simulink model "Convolution_Ex2"  (R2025a)
settings: Solver=VariableStepAuto  StartTime=0.0  StopTime=128/100e6  RelTol=1e-3
undefined symbols (not defined in the file): S, Same, vsva2197, xcvc1902
libraries: aieDSP x1, vmcUtilities x1
settings Model: Creator=sdegala  LastModifiedBy=robg
settings ModelReferenceCC: EnableRefExpFcnMdlSchedulingChecks=on
settings RTWCC: GPUComputeCapability=3.5

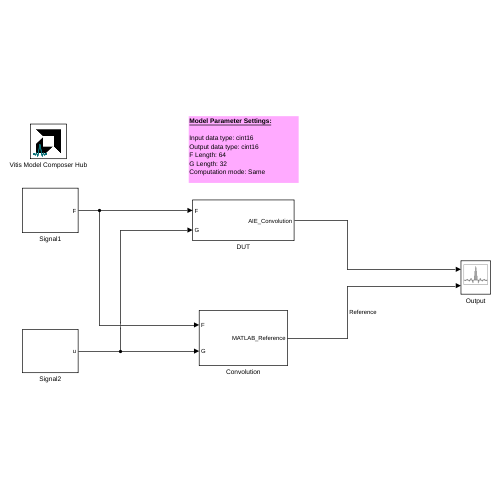
[thumbnail: Simulink's stored preview of the top-level diagram]
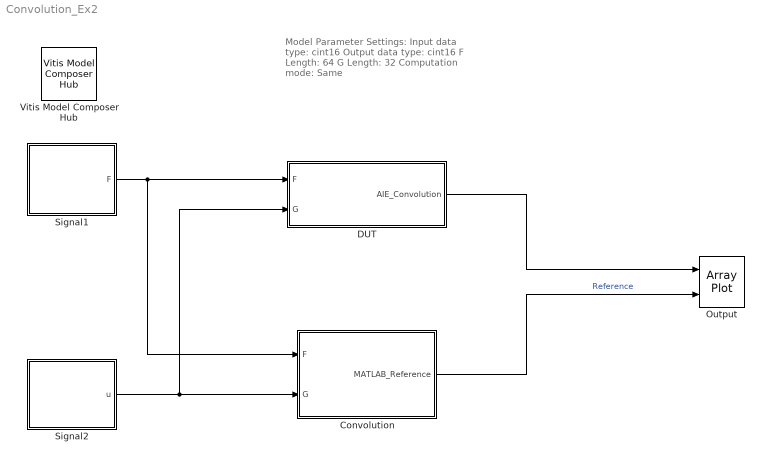
== system Convolution_Ex2 ==
  note: Model Parameter Settings:
      |
      | Input data type: cint16
      | Output data type: cint16
      | F Length: 64
      | G Length: 32
      | Computation mode: Same
  Convolution : Subsystem
  DUT : Subsystem
  Output : ArrayPlot  NumInputPorts=2  WindowPosition=[568.000000,395.000000,800.000000,500.000000,]  Visible=on  ScopeFrameLocation=window  YLimits=[-6.75 60.75]  ShowLegend=on
  Signal1 : Subsystem
  Signal2 : Subsystem
  Vitis Model Composer Hub : vmcUtilities/Vitis Model Composer Hub  Tag=genX  CodeGeneration=off  StartColumn=1  NumberOfColumns=1  TargetDirectory=./code  exportDesign=off  analyzeDesign=off  validateDesignOnHw=off  ExportType=AI Engines  IpVendor=xilinx.com  IpLibrary=hls  IpVersion=1.0  IpHWLanguage=Verilog  AieCompilerOptions={}  AieSimulatorOptions={}  CreateTestbench=off  TestbenchStackSize=10  RunRtlSim=off  RunCSim=off  RunAieSim=off  enableSimulationTimeout=on  enableGraphIterations=on  AieSimTimeout=50000  AieGraphIterations=-1  RunAieSimProfiling=off  LaunchVitisAnalyzer=off  PlotOutput=off  RunX86Sim=off  X86SimTimeout=10  GenHwImage=off  GenLibadfXo=off  GenHwValidationCode=off  PlatformType=Not Specified  HwSystemType=Baremetal  HwValidationTarget=hw  ProjDevice=xcvc1902-vsva2197-1LP-e-S  ProjDevicePart=xcvc1902-vsva2197-1LP-e-S  AIEType=AIE  SamplePeriod=-1  ClockFrequency=200  DataPathParallelism=1  xilinxfamily=versalaicore  part=xcvc1902  speed=-1LP-e-S  package=vsva2197  directory=./netlist  testbench=off  incr_netlist=off  synthesis_tool=Vivado  clock_wrapper=Clock Enables  dbl_ovrd=According to Block Masks  dcm_input_clock_period=10  sysclk_period=10  simulink_period=1  eval_field=0  LogFileName=''  NThreads=4
  wires:
  Signal2/1(u) -> DUT/2(G), Convolution/2(G)
  DUT/1(AIE_Convolution) -> Output/1
  Signal1/1(F) -> DUT/1(F), Convolution/1(F)
  Convolution/1(MATLAB_Reference) -> Output/2  "Reference"

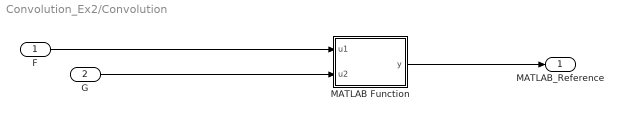
== system Convolution_Ex2/Convolution ==
  F : Inport
  G : Inport  Port=2
  MATLAB Function : MATLAB Function  TreatAsAtomicUnit=on
  MATLAB_Reference : Outport
  wires:
  F/1 -> MATLAB Function/1(u1)
  MATLAB Function/1(y) -> MATLAB_Reference/1
  G/1 -> MATLAB Function/2(u2)

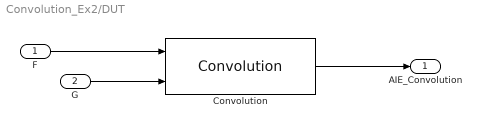
== system Convolution_Ex2/DUT ==
  F : Inport
  G : Inport  Port=2
  Convolution : aieDSP/Convolution  AIE_VARIANT=1  api=0  data_type_f=cint16  data_type_g=cint16  data_type_out=cint16  function_type=1  compute_mode=Same (1)  f_sample_size=64  g_sample_size=32  USE_RTP_VECTOR_LENGTHS=off  num_frames=1  shift_output=0  rnd_mode=Floor  sat_mode=None  no_of_kernels=1  casc_length=1  blockJsonConstraints=[]  blockJsonConstraintsInternal=[]  spec=vmc_conv.json  SerializedMaskParamNames=[]  SerializedMaskParamValues=[]  SerializedMaskParamVisibilities=[]  block_type=Convolution  SerializedMaskParamDataypes=uint|uint|typename|typename|typename|uint|uint|uint|uint|uint|uint|uint|uint|uint|uint|uint  SerializedMaskParamEnumStrArr=0|0|0|0|0|0|Full (0),Same (1),Valid (2)|0|0|0|0|0|Floor,Ceiling,Round to positive infinity,Round to negative infinity,Round symmetrical to infinity,Round symmetrical to zero,Round convergent to even,Round convergent to odd|None,Saturate,Symmetric|0|0  SerializedMaskParamEnumValArr=0|0|0|0|0|0|0,1,2|0|0|0|0|0|0,1,2,3,4,5,6,7|0,1,3|0|0  SerializedMaskParamVectorArr=0|0|0|0|0|0|0|0|0|0|0|0|0|0|0|0  SerializedMaskParamKeys=AIE_VARIANT|TP_API|TT_DATA_F|TT_DATA_G|TT_DATA_OUT|TP_FUNCT_TYPE|TP_COMPUTE_MODE|TP_F_LEN|TP_G_LEN|TP_USE_RTP_VECTOR_LENGTHS|TP_NUM_FRAMES|TP_SHIFT|TP_RND|TP_SAT|TP_PHASES|TP_CASC_LEN
  AIE_Convolution : Outport
  wires:
  F/1 -> Convolution/1
  G/1 -> Convolution/2
  Convolution/1 -> AIE_Convolution/1

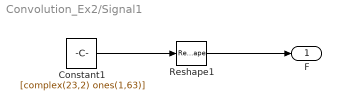
== system Convolution_Ex2/Signal1 ==
  Constant1 : Constant  Value=[complex(23,2) ones(1,63)]  OutDataTypeStr=int16  SampleTime=1/100e6
  Reshape1 : Reshape
  F : Outport
  wires:
  Reshape1/1 -> F/1
  Constant1/1 -> Reshape1/1

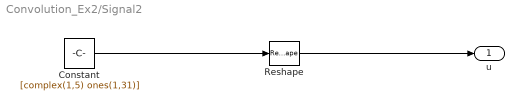
== system Convolution_Ex2/Signal2 ==
  Constant : Constant  Value=[complex(1,5) ones(1,31)]  OutDataTypeStr=int16  SampleTime=1/100e6
  Reshape : Reshape
  u : Outport
  wires:
  Reshape/1 -> u/1
  Constant/1 -> Reshape/1

== matlab function Convolution_Ex2/Convolution/MATLAB Function ==
  data: u1 input; y output; u2 input
function y = func(u1,u2)

y = int16(conv(u1,u2,'same'));
